simulink model "my_gm_HDLPayloadFull"  (R2024a)
settings: Solver=FixedStepDiscrete  StartTime=0.0  StopTime=stopTime  RelTol=1e-3
values from neighbouring files (symbols this model uses):
  pWords = [pWords binl2str(pBitsRaw{i})]    [testPayloadFull.m]
undefined symbols (not defined in the file or in its folder): fs, msgIn
libraries: hdlmdlgenlib x66, hdlsllib x16, dspsrcs4 x9, dspsigops x9, simulink x4, whdlutilities x4, whdledac x1
(part 2 of 2)

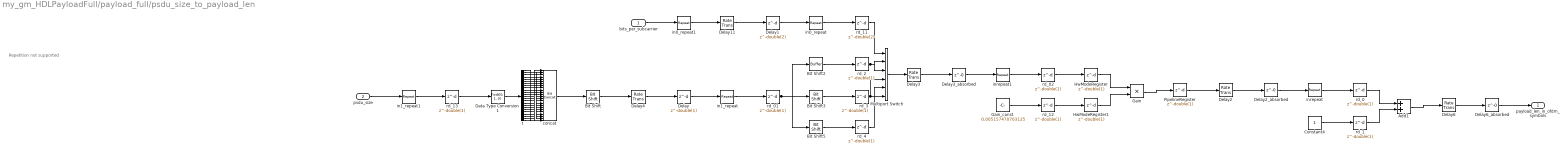
== system my_gm_HDLPayloadFull/payload_full/psdu_size_to_payload_len ==
  note: Repetition not supported
  bits_per_subcarrier : Inport  OutDataTypeStr=fixdt(0, 4, 0)  PortDimensions=1  SampleTime=8e-08
  psdu_size : Inport  Port=2  OutDataTypeStr=boolean  PortDimensions=[24]  SampleTime=8e-08
  Add1 : Sum  OutDataTypeStr=uint16  AccumDataTypeStr=fixdt(0, 17, 0)  SampleTime=1e-08
  Bit Shift : hdlsllib/Logic and Bit Operations/Bit Shift  mode=Shift Left Logical  N=double(4)
  Bit Shift2 : hdlmdlgenlib/Buffer
  Bit Shift3 : hdlsllib/Logic and Bit Operations/Bit Shift  mode=Shift Right Arithmetic  N=double(1)
  Bit Shift5 : hdlsllib/Logic and Bit Operations/Bit Shift  mode=Shift Right Arithmetic  N=double(4)
  Constant4 : Constant  OutDataTypeStr=fixdt(0, 1, 0)  SampleTime=1e-08
  Data Type Conversion1 : DataTypeConversion  OutDataTypeStr=fixdt(0, 1, 0)  SampleTime=1e-08  SaturateOnIntegerOverflow=off  RndMeth=Floor
  Delay : Delay  DelayLength=double(1)  InitialCondition=0  SampleTime=8e-08
  Delay1 : Delay  DelayLength=double(2)  InitialCondition=0  SampleTime=8e-08
  Delay{2..4,6,11} (5 alike) : RateTransition  OutPortSampleTimeOpt=Multiple of input port sample time  OutPortSampleTimeMultiple=8
  Delay2_absorbed : Delay  DelayLength=0
  Delay3_absorbed : Delay  DelayLength=0
  Delay6_absorbed : Delay  DelayLength=0
  Gain : Product  Inputs=**  OutDataTypeStr=uint16  SampleTime=1e-08
  Gain_const : Constant  Value=0.005157470703125  OutDataTypeStr=fixdt(1, 16, 15)  SampleTime=1e-08
  HwModeRegister : Delay  DelayLength=double(1)  InitialCondition=0  SampleTime=1e-08
  HwModeRegister1 : Delay  DelayLength=double(1)  InitialCondition=0  SampleTime=1e-08
  Multiport Switch : MultiPortSwitch  DataPortOrder=Zero-based contiguous  Inputs=5  DiagnosticForDefault=None  zeroidx=on  OutDataTypeStr=fixdt(0, 24, 0)  SampleTime=1e-08  SaturateOnIntegerOverflow=off  InputSameDT=off
  PipelineRegister : Delay  DelayLength=double(1)  InitialCondition=0  SampleTime=1e-08
  concat : hdlsllib/Logic and Bit Operations/Bit Concat  numInputs=24
  in0_repeat : dspsigops/Repeat  FactorSource=Dialog parameter  N=double(8)  Nmax=16  RateOptions=Allow multirate processing  ic=0  mode=Unused parameter value
  in0_repeat1 : dspsigops/Repeat  FactorSource=Dialog parameter  N=double(8)  Nmax=16  RateOptions=Allow multirate processing  ic=0  mode=Unused parameter value
  in1_repeat : dspsigops/Repeat  FactorSource=Dialog parameter  N=double(8)  Nmax=16  RateOptions=Allow multirate processing  ic=0  mode=Unused parameter value
  in1_repeat1 : dspsigops/Repeat  FactorSource=Dialog parameter  N=double(8)  Nmax=16  RateOptions=Allow multirate processing  ic=0  mode=Unused parameter value
  inrepeat : dspsigops/Repeat  FactorSource=Dialog parameter  N=double(8)  Nmax=16  RateOptions=Allow multirate processing  ic=0  mode=Unused parameter value
  inrepeat1 : dspsigops/Repeat  FactorSource=Dialog parameter  N=double(8)  Nmax=16  RateOptions=Allow multirate processing  ic=0  mode=Unused parameter value
  rd_{0..4,12..13} (7 alike) : Delay  DelayLength=double(1)  InitialCondition=0  SampleTime=1e-08
  rd_01 : Delay  DelayLength=double(1)  InitialCondition=0  SampleTime=1e-08
  rd_02 : Delay  DelayLength=double(1)  InitialCondition=0  SampleTime=1e-08
  rd_11 : Delay  DelayLength=double(2)  InitialCondition=0  SampleTime=1e-08
  t : Demux  Outputs=24
  payload_len_in_ofdm_symbols : Outport  SampleTime=8e-08
  wires:
  bits_per_subcarrier/1 -> in0_repeat1/1
  psdu_size/1 -> in1_repeat1/1
  Delay1/1 -> in0_repeat/1
  Delay/1 -> in1_repeat/1
  inrepeat/1 -> rd_0/1
  Delay6/1 -> Delay6_absorbed/1
  Delay6_absorbed/1 -> payload_len_in_ofdm_symbols/1
  in0_repeat/1 -> rd_11/1
  in1_repeat/1 -> rd_01/1
  Multiport Switch/1 -> Delay3/1
  Delay3/1 -> Delay3_absorbed/1
  Delay3_absorbed/1 -> inrepeat1/1
  inrepeat1/1 -> rd_02/1
  PipelineRegister/1 -> Delay2/1
  Delay2/1 -> Delay2_absorbed/1
  Delay2_absorbed/1 -> inrepeat/1
  Delay11/1 -> Delay1/1
  in0_repeat1/1 -> Delay11/1
  in1_repeat1/1 -> rd_13/1
  Bit Shift/1 -> Delay4/1
  Delay4/1 -> Delay/1
  Constant4/1 -> rd_1/1
  Add1/1 -> Delay6/1
  rd_1/1 -> Add1/2
  rd_0/1 -> Add1/1
  Bit Shift5/1 -> rd_4/1
  rd_11/1 -> Multiport Switch/1
  rd_4/1 -> Multiport Switch/6
  Bit Shift3/1 -> rd_3/1
  rd_3/1 -> Multiport Switch/4, Multiport Switch/5
  Bit Shift2/1 -> rd_2/1
  rd_2/1 -> Multiport Switch/2, Multiport Switch/3
  rd_01/1 -> Bit Shift2/1, Bit Shift5/1, Bit Shift3/1
  Gain_const/1 -> rd_12/1
  rd_12/1 -> HwModeRegister1/1
  rd_02/1 -> HwModeRegister/1
  Data Type Conversion1/1 -> t/1
  concat/1 -> Bit Shift/1
  t/1 -> concat/24
  t/2 -> concat/23
  t/3 -> concat/22
  t/4 -> concat/21
  t/5 -> concat/20
  t/6 -> concat/19
  t/7 -> concat/18
  t/8 -> concat/17
  t/9 -> concat/16
  t/10 -> concat/15
  t/11 -> concat/14
  t/12 -> concat/13
  t/13 -> concat/12
  t/14 -> concat/11
  t/15 -> concat/10
  t/16 -> concat/9
  t/17 -> concat/8
  t/18 -> concat/7
  t/19 -> concat/6
  t/20 -> concat/5
  t/21 -> concat/4
  t/22 -> concat/3
  t/23 -> concat/2
  t/24 -> concat/1
  rd_13/1 -> Data Type Conversion1/1
  Gain/1 -> PipelineRegister/1
  HwModeRegister/1 -> Gain/1
  HwModeRegister1/1 -> Gain/2

== system my_gm_HDLPayloadFull/payload_full/puncturer ==
  data_in : Inport  OutDataTypeStr=boolean  SampleTime=1e-08
  ctrl_in : Inport  Port=2  SampleTime=1e-08
  data_out : Outport  SampleTime=1e-08
  ctrl_out : Outport  Port=2  SampleTime=1e-08
  wires:
  data_in/1 -> data_out/1
  ctrl_in/1 -> ctrl_out/1

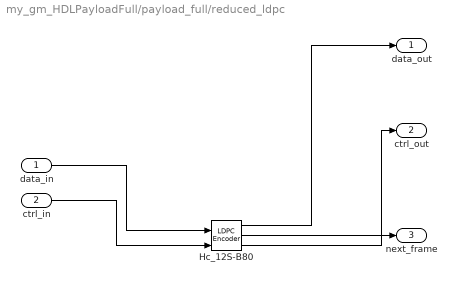
== system my_gm_HDLPayloadFull/payload_full/reduced_ldpc ==
  data_in : Inport  OutDataTypeStr=boolean  SampleTime=1e-08
  ctrl_in : Inport  Port=2  SampleTime=1e-08
  Hc_12S-B80 : whdledac/LDPC Encoder  ParityCheckMatrix=Hc_12S  BlockSize=80  SimulateUsing=Code generation
  data_out : Outport  SampleTime=1e-08
  ctrl_out : Outport  Port=2  SampleTime=1e-08
  next_frame : Outport  Port=3  SampleTime=1e-08
  wires:
  data_in/1 -> Hc_12S-B80/1
  ctrl_in/1 -> Hc_12S-B80/2
  Hc_12S-B80/1 -> data_out/1
  Hc_12S-B80/2 -> ctrl_out/1
  Hc_12S-B80/3 -> next_frame/1

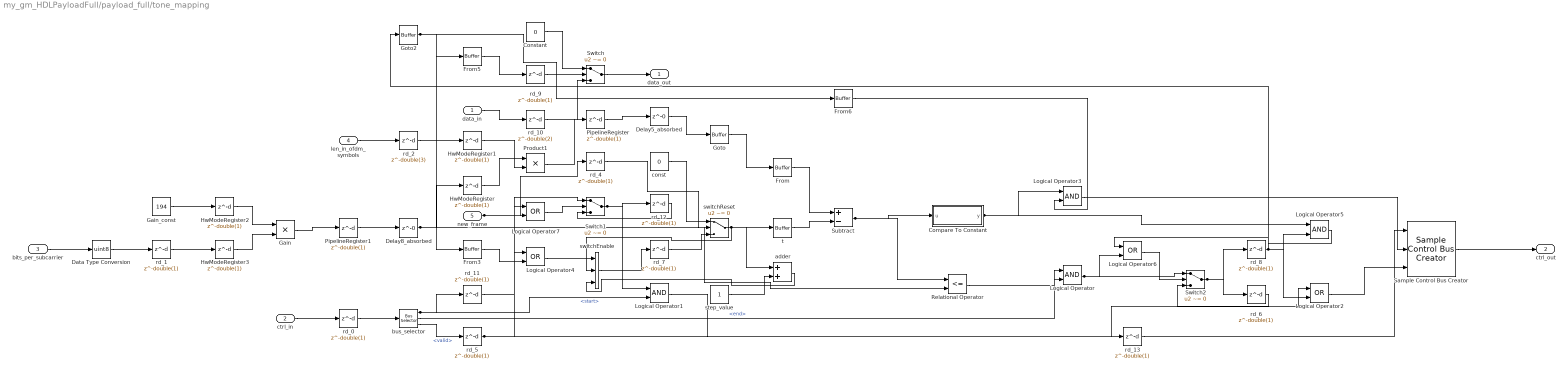
== system my_gm_HDLPayloadFull/payload_full/tone_mapping ==
  data_in : Inport  OutDataTypeStr=boolean  PortDimensions=1  SampleTime=1e-08
  ctrl_in : Inport  Port=2
  bits_per_subcarrier : Inport  Port=3  OutDataTypeStr=fixdt(0, 4, 0)  PortDimensions=1  SampleTime=1e-08
  len_in_ofdm_symbols : Inport  Port=4  OutDataTypeStr=uint16  PortDimensions=1  SampleTime=1e-08
  new_frame : Inport  Port=5  OutDataTypeStr=boolean  PortDimensions=1  SampleTime=1e-08
  Compare To Constant : Subsystem  mask(Compare To Constant){relop===, const=double(1), OutDataTypeStr=boolean, ZeroCross=on}
      mask prompts: relop "Simulink:masks:Operator_MP"; const "Simulink:masks:ConstantValue_MP"; OutDataTypeStr "Simulink:masks:OutputDataType_MP"; ZeroCross "Simulink:masks:EnableZerocrossingDetection_MP"
      mask help: Simulink:masks:CompareToConstant_MD
      mask init:
      | OutDataTypeStr = 'boolean';
      | ZeroCross = 'on';
      | blkName = 'HDLPayloadFull/payload_full/tone_mapping/Compare\nTo Constant';
      | const = double(1);
      | const_str = '1';
      | const_val = double(1);
      | relop = '==';
      | setValue = 'boolean';
      | str = '== 1';
      mask TypeOptions relop: == | ~= | < | <= | >= | >
      mask TypeOptions OutDataTypeStr: Simulink:masks:uint8 | Simulink:masks:boolean
      mask Callback ZeroCross: sl('zeroCrossEnable', gcbh);
      mask Display: disp(str)
  Constant : Constant  Value=0  OutDataTypeStr=boolean  SampleTime=1e-08
  Data Type Conversion : DataTypeConversion  OutDataTypeStr=uint8  SampleTime=1e-08  SaturateOnIntegerOverflow=off  RndMeth=Floor
  Delay5_absorbed : Delay  DelayLength=0
  Delay8_absorbed : Delay  DelayLength=0
  From{,3,5..6} (4 alike) : hdlmdlgenlib/Buffer
  Gain : Product  Inputs=**  OutDataTypeStr=fixdt(0, 10, 0)  SampleTime=1e-08
  Gain_const : Constant  Value=194  OutDataTypeStr=uint8  SampleTime=1e-08
  Goto : hdlmdlgenlib/Buffer
  Goto2 : hdlmdlgenlib/Buffer
  HwModeRegister{,1..3} (4 alike) : Delay  DelayLength=double(1)  InitialCondition=0  SampleTime=1e-08
  Logical Operator{,1,3,5} (4 alike) : Logic  AllPortsSameDT=off  OutDataTypeStr=boolean  SampleTime=1e-08
  Logical Operator{2,4,6..7} (4 alike) : Logic  Operator=OR  AllPortsSameDT=off  OutDataTypeStr=boolean  SampleTime=1e-08
  PipelineRegister : Delay  DelayLength=double(1)  InitialCondition=0  SampleTime=1e-08
  PipelineRegister1 : Delay  DelayLength=double(1)  InitialCondition=0  SampleTime=1e-08
  Product1 : Product  Inputs=**  OutDataTypeStr=fixdt(0, 26, 0)  SampleTime=1e-08
  Relational Operator : RelationalOperator  Operator=<=  OutDataTypeStr=boolean  SampleTime=1e-08  InputSameDT=off
  Sample Control Bus Creator : whdlutilities/Sample Control Bus Creator
  Subtract : Sum  Inputs=+-  OutDataTypeStr=fixdt(0, 26, 0)  AccumDataTypeStr=fixdt(1, 33, 0)  SampleTime=1e-08
  Switch : Switch  Criteria=u2 ~= 0  Threshold=double(0)  OutDataTypeStr=boolean  SampleTime=1e-08  SaturateOnIntegerOverflow=off  InputSameDT=off
  Switch1 : Switch  Criteria=u2 ~= 0  Threshold=double(0)  OutDataTypeStr=boolean  SampleTime=1e-08  SaturateOnIntegerOverflow=off  InputSameDT=off
  Switch2 : Switch  Criteria=u2 ~= 0  Threshold=double(0)  OutDataTypeStr=boolean  SampleTime=1e-08  SaturateOnIntegerOverflow=off  InputSameDT=off
  adder : Sum  OutDataTypeStr=uint32  AccumDataTypeStr=uint32  SampleTime=1e-08
  bus_selector : BusSelector  OutputSignals=start,end,valid
  const : Constant  Value=0  VectorParams1D=off  OutDataTypeStr=uint32  SampleTime=1e-08
  rd_{0..1,4..9,11..13} (11 alike) : Delay  DelayLength=double(1)  InitialCondition=0  SampleTime=1e-08
  rd_10 : Delay  DelayLength=double(2)  InitialCondition=0  SampleTime=1e-08
  rd_2 : Delay  DelayLength=double(3)  InitialCondition=0  SampleTime=1e-08
  step_value : Constant  VectorParams1D=off  OutDataTypeStr=uint32  SampleTime=1e-08
  switchEnable : MultiPortSwitch  DataPortOrder=Zero-based contiguous  Inputs=2  DiagnosticForDefault=None  zeroidx=on  OutDataTypeStr=uint32  SampleTime=1e-08  SaturateOnIntegerOverflow=off  InputSameDT=off
  switchReset : Switch  Criteria=u2 ~= 0  Threshold=double(0)  OutDataTypeStr=uint32  SampleTime=1e-08  SaturateOnIntegerOverflow=off  InputSameDT=off
  t : hdlmdlgenlib/Buffer
  data_out : Outport  SampleTime=1e-08
  ctrl_out : Outport  Port=2
  wires:
  data_in/1 -> rd_10/1
  ctrl_in/1 -> rd_0/1
  bits_per_subcarrier/1 -> Data Type Conversion/1
  len_in_ofdm_symbols/1 -> rd_2/1
  new_frame/1 -> rd_4/1, Logical Operator7/2, Switch1/1
  Compare To Constant/1(y) -> Logical Operator3/1, Logical Operator5/1
  Constant/1 -> Switch/1
  Data Type Conversion/1 -> rd_1/1
  Delay5_absorbed/1 -> Goto/1
  Delay8_absorbed/1 -> Relational Operator/2, HwModeRegister/1
  From/1 -> Subtract/1
  From5/1 -> rd_9/1
  From6/1 -> Logical Operator3/2
  Logical Operator1/1 -> rd_13/1
  Logical Operator2/1 -> Sample Control Bus Creator/3
  Logical Operator3/1 -> Sample Control Bus Creator/2
  Sample Control Bus Creator/1 -> ctrl_out/1
  bus_selector/1 -> rd_11/1, Logical Operator1/2  "<start>"
  bus_selector/2 -> Logical Operator/1  "<end>"
  Switch/1 -> data_out/1
  Switch1/1 -> rd_12/1, Logical Operator1/1
  Goto/1 -> From/1
  Goto2/1 -> From6/1, From5/1, From3/1
  Gain_const/1 -> HwModeRegister2/1
  step_value/1 -> adder/2
  const/1 -> switchReset/1
  switchReset/1 -> t/1, adder/1, switchEnable/2
  adder/1 -> switchEnable/3
  From3/1 -> Logical Operator4/2
  Logical Operator4/1 -> switchEnable/1
  switchEnable/1 -> rd_7/1
  Switch2/1 -> rd_6/1, rd_8/1
  Logical Operator5/1 -> Logical Operator6/1
  Logical Operator6/1 -> Switch2/2
  Relational Operator/1 -> Logical Operator/2
  Logical Operator/1 -> Switch2/1, Logical Operator6/2
  t/1 -> Subtract/2
  Subtract/1 -> Relational Operator/1, Compare To Constant/1(u)
  Logical Operator7/1 -> Switch1/2
  PipelineRegister/1 -> Delay5_absorbed/1
  PipelineRegister1/1 -> Delay8_absorbed/1
  rd_10/1 -> Switch/3
  rd_0/1 -> bus_selector/1
  rd_2/1 -> HwModeRegister1/1
  rd_4/1 -> switchReset/2
  rd_1/1 -> HwModeRegister3/1
  rd_13/1 -> Sample Control Bus Creator/1
  rd_11/1 -> Logical Operator7/1
  rd_7/1 -> switchReset/3
  rd_6/1 -> Switch2/3
  rd_12/1 -> Switch1/3
  rd_9/1 -> Switch/2
  rd_8/1 -> Goto2/1, Logical Operator5/2, Logical Operator2/2
  bus_selector/3 -> rd_5/1  "<valid>"
  rd_5/1 -> Logical Operator4/1, Logical Operator2/1
  Product1/1 -> PipelineRegister/1
  HwModeRegister/1 -> Product1/1
  HwModeRegister1/1 -> Product1/2
  Gain/1 -> PipelineRegister1/1
  HwModeRegister2/1 -> Gain/1
  HwModeRegister3/1 -> Gain/2

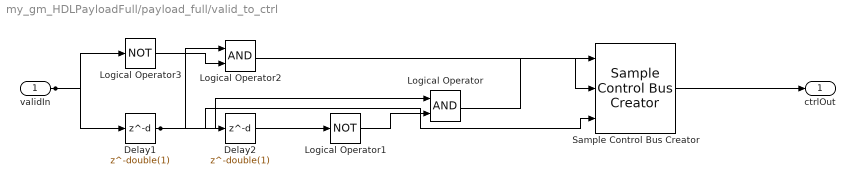
== system my_gm_HDLPayloadFull/payload_full/valid_to_ctrl ==
  validIn : Inport  OutDataTypeStr=boolean  SampleTime=1e-08
  Delay1 : Delay  DelayLength=double(1)  InitialCondition=0  SampleTime=1e-08
  Delay2 : Delay  DelayLength=double(1)  InitialCondition=0  SampleTime=1e-08
  Logical Operator : Logic  AllPortsSameDT=off  OutDataTypeStr=boolean  SampleTime=1e-08
  Logical Operator1 : Logic  Operator=NOT  Inputs=1  AllPortsSameDT=off  OutDataTypeStr=boolean  SampleTime=1e-08
  Logical Operator2 : Logic  AllPortsSameDT=off  OutDataTypeStr=boolean  SampleTime=1e-08
  Logical Operator3 : Logic  Operator=NOT  Inputs=1  AllPortsSameDT=off  OutDataTypeStr=boolean  SampleTime=1e-08
  Sample Control Bus Creator : whdlutilities/Sample Control Bus Creator
  ctrlOut : Outport  SampleTime=1e-08
  wires:
  validIn/1 -> Logical Operator3/1, Delay1/1
  Delay1/1 -> Logical Operator2/1, Logical Operator/1, Delay2/1, Sample Control Bus Creator/3
  Delay2/1 -> Logical Operator1/1
  Logical Operator/1 -> Sample Control Bus Creator/1
  Logical Operator1/1 -> Logical Operator/2
  Logical Operator2/1 -> Sample Control Bus Creator/2
  Logical Operator3/1 -> Logical Operator2/2
  Sample Control Bus Creator/1 -> ctrlOut/1

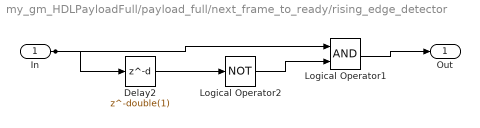
== system my_gm_HDLPayloadFull/payload_full/next_frame_to_ready/rising_edge_detector ==
  In : Inport  OutDataTypeStr=boolean  SampleTime=8e-08
  Delay2 : Delay  DelayLength=double(1)  InitialCondition=0  SampleTime=8e-08
  Logical Operator1 : Logic  AllPortsSameDT=off  OutDataTypeStr=boolean  SampleTime=8e-08
  Logical Operator2 : Logic  Operator=NOT  Inputs=1  AllPortsSameDT=off  OutDataTypeStr=boolean  SampleTime=8e-08
  Out : Outport  SampleTime=8e-08
  wires:
  In/1 -> Logical Operator1/1, Delay2/1
  Logical Operator1/1 -> Out/1
  Delay2/1 -> Logical Operator2/1
  Logical Operator2/1 -> Logical Operator1/2

== system my_gm_HDLPayloadFull/payload_full/tone_mapping/Compare To Constant ==
  u : Inport  OutDataTypeStr=fixdt(0, 26, 0)  SampleTime=1e-08
  Compare : RelationalOperator  Operator===  OutDataTypeStr=boolean  SampleTime=1e-08
  Constant : Constant  OutDataTypeStr=fixdt(0, 26, 0)  SampleTime=1e-08
  y : Outport  SampleTime=1e-08
  wires:
  u/1 -> Compare/1
  Compare/1 -> y/1
  Constant/1 -> Compare/2
